simulink model "flowchart"  (R2020a)
settings: Solver=VariableStepAuto  StartTime=0.0  StopTime=5  RelTol=1e-3
settings Model: Creator=I3  LastModifiedBy=I3

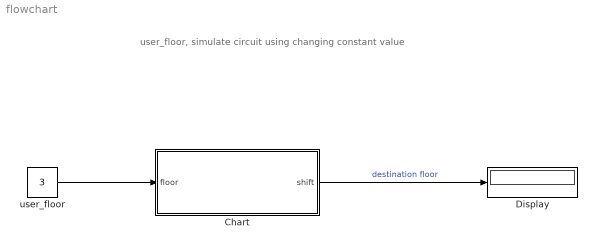
== system flowchart ==
  note: user_floor, simulate circuit using changing constant value
  Chart : Stateflow chart  TreatAsAtomicUnit=on
  Display : Display
  user_floor : Constant  Value=3
  wires:
  user_floor/1 -> Chart/1(floor)
  Chart/1(shift) -> Display/1  "destination floor"

== stateflow chart flowchart/Chart ==
  (default) -> (junction 3) : {current =0;shift=0;}
  (junction 14) -> (junction 3) [order 1] : [current~=floor]
  (junction 3) -> (junction 5) [order 1] : [current<=floor && floor<6]
  (junction 3) -> (junction 6) [order 2]
  (junction 5) -> (junction 16) : {current=current+1;}
  (junction 6) -> (junction 12) [order 1] : [current>=floor && floor<6]
  (junction 6) -> (junction 14) [order 2] : {current=0;}
  (junction 12) -> (junction 15) : {current = current -1;}
  (junction 15) -> (junction 14)
  (junction 16) -> (junction 15)
  (junction 14) -> (junction 17) [order 2] : {shift =current;}
  data: floor input; shift output; current local =0
